simulink model "system_ID"  (R2023b)
settings: Solver=ode4  StartTime=0.0  StopTime=70  FixedStep=0.001  RelTol=1e-3
values from neighbouring files (symbols this model uses):
  Fc = 0.00040    (= 0.0004)    [MPC_casadi_block.m]    (also in continuous_cartpend.m; init_HAC_simulation.m; init_MPC.m; init_NMPC.m)
  g = [g; st_next - st_next_RK4]    [MPC_cartPend_casadi.m]    (also in MPC_cartPend_casadi_scaled.m; MPC_casadi_block.m; continuous_cartpend.m = 9.80665; init_HAC_simulation.m = 9.80665)
  I = 8.7395e-04    (= 0.00087395)    [MPC_casadi_block.m]    (also in continuous_cartpend.m = 0.0008739525; init_HAC_simulation.m = 0.0008739525; init_MPC.m = 0.0008739525; init_NMPC.m = 0.0008739525)
  init_angle = 180    [MPC_cartPend_casadi.m]    (also in init_HAC_simulation.m = deg2rad(initial_angle); init_MPC.m = -0.349065850399; init_NMPC.m = 3.14159265359; init_PID_cartpole.m = 0)
  kd = 0.000161    [MPC_casadi_block.m]    (also in continuous_cartpend.m; init_HAC_simulation.m; init_MPC.m; init_NMPC.m)
  kdr = 0.000001    (= 1e-06)    [MPC_casadi_block.m]    (also in continuous_cartpend.m; init_HAC_simulation.m; init_MPC.m; init_NMPC.m)
  kt = 150    [MPC_casadi_block.m]    (also in continuous_cartpend.m; init_HAC_simulation.m; init_MPC.m; init_NMPC.m)
  L = 0.1500    (= 0.15)    [MPC_casadi_block.m]    (also in continuous_cartpend.m; init_HAC_simulation.m; init_MPC.m; init_NMPC.m)
  m = 0.116527    [MPC_casadi_block.m]    (also in continuous_cartpend.m; init_HAC_simulation.m; init_MPC.m; init_NMPC.m)
libraries: simulink_extras x1
settings Model: Creator=doann  LastModifiedBy=doann
settings OptimizationCC: ReuseModelBlockBuffer=off

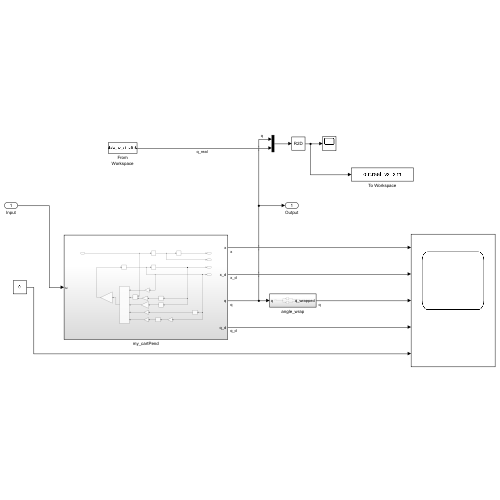
[thumbnail: Simulink's stored preview of the top-level diagram]
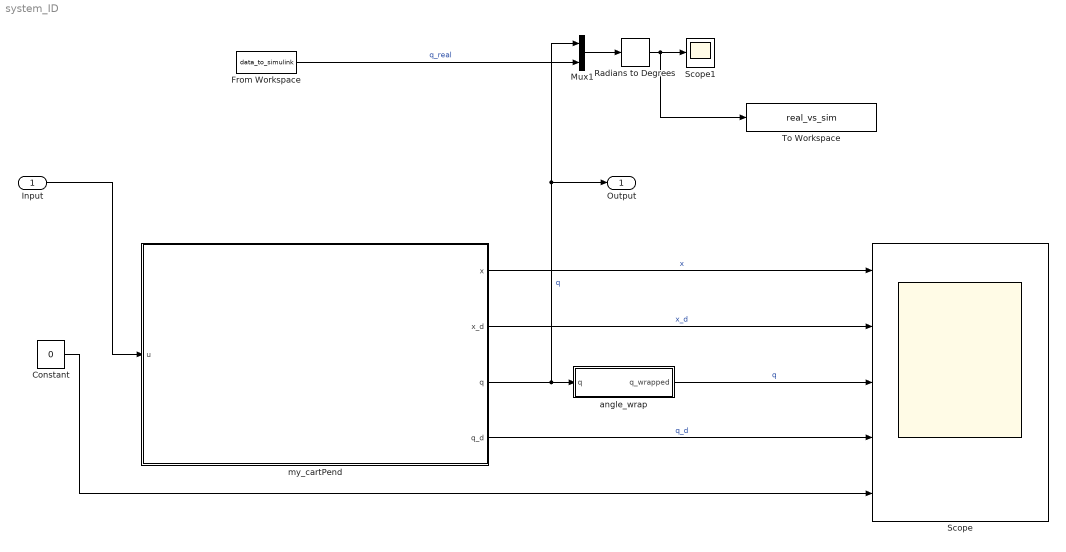
== system system_ID ==
  Input : Inport
  Constant : Constant  Value=0
  From Workspace : FromWorkspace  VariableName=data_to_simulink  OutputAfterFinalValue=Holding final value
  Mux1 : Mux  Inputs=2
  Radians to Degrees : simulink_extras/Transformations/Radians to Degrees
  Scope : Scope  NumInputPorts=5
  Scope1 : Scope
  To Workspace : ToWorkspace  VariableName=real_vs_sim  SaveFormat=Structure With Time  SampleTime=-1
  angle_wrap : Subsystem
  my_cartPend : Subsystem
  Output : Outport
  wires:
  Mux1/1 -> Radians to Degrees/1
  From Workspace/1 -> Mux1/2  "q_real"
  my_cartPend/3(q) -> Mux1/1, Output/1, angle_wrap/1(q)  "q"
  Constant/1 -> Scope/5
  angle_wrap/1(q_wrapped) -> Scope/3  "q"
  my_cartPend/1(x) -> Scope/1  "x"
  my_cartPend/2(x_d) -> Scope/2  "x_d"
  my_cartPend/4(q_d) -> Scope/4  "q_d"
  Input/1 -> my_cartPend/1(u)
  Radians to Degrees/1 -> To Workspace/1, Scope1/1

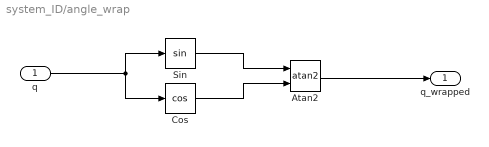
== system system_ID/angle_wrap ==
  q : Inport
  Atan2 : Trigonometry  Operator=atan2
  Cos : Trigonometry  Operator=cos
  Sin : Trigonometry
  q_wrapped : Outport
  wires:
  Cos/1 -> Atan2/2
  q/1 -> Sin/1, Cos/1
  Sin/1 -> Atan2/1
  Atan2/1 -> q_wrapped/1

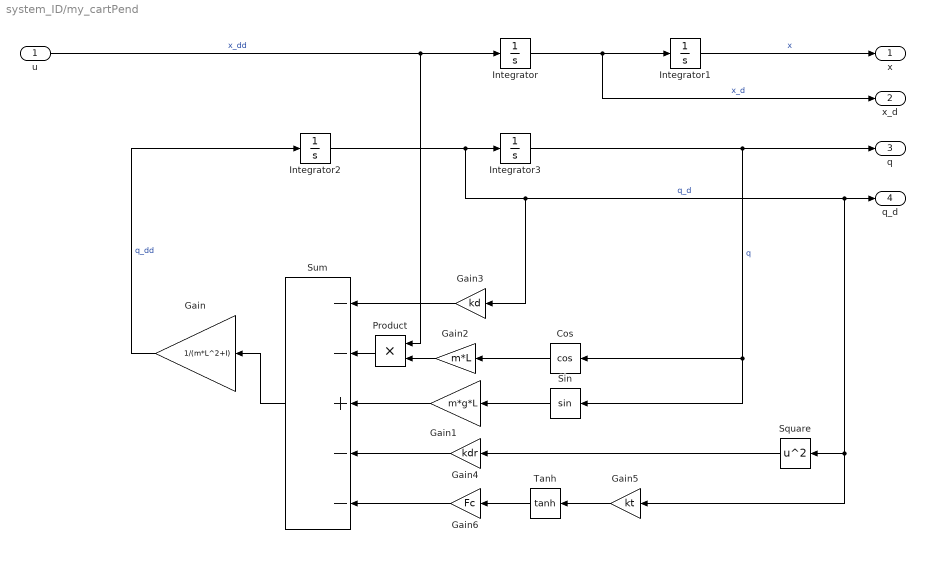
== system system_ID/my_cartPend ==
  u : Inport
  Cos : Trigonometry  Operator=cos
  Gain : Gain  Gain=1/(m*L^2+I)
  Gain1 : Gain  Gain=m*g*L
  Gain2 : Gain  Gain=m*L
  Gain3 : Gain  Gain=kd
  Gain4 : Gain  Gain=kdr
  Gain5 : Gain  Gain=kt
  Gain6 : Gain  Gain=Fc
  Integrator : Integrator
  Integrator1 : Integrator
  Integrator2 : Integrator
  Integrator3 : Integrator  InitialCondition=init_angle
  Product : Product
  Sin : Trigonometry
  Square : Math  Operator=square
  Sum : Sum  Inputs=--+--
  Tanh : Trigonometry  Operator=tanh
  x : Outport
  x_d : Outport  Port=2
  q : Outport  Port=3
  q_d : Outport  Port=4
  wires:
  u/1 -> Product/1, Integrator/1  "x_dd"
  Integrator/1 -> x_d/1, Integrator1/1  "x_d"
  Integrator1/1 -> x/1  "x"
  Integrator3/1 -> Sin/1, Cos/1, q/1  "q"
  Integrator2/1 -> Gain3/1, Gain5/1, Square/1, q_d/1, Integrator3/1  "q_d"
  Sin/1 -> Gain1/1
  Cos/1 -> Gain2/1
  Sum/1 -> Gain/1
  Gain/1 -> Integrator2/1  "q_dd"
  Gain1/1 -> Sum/3
  Gain3/1 -> Sum/1
  Gain2/1 -> Product/2
  Product/1 -> Sum/2
  Square/1 -> Gain4/1
  Tanh/1 -> Gain6/1
  Gain5/1 -> Tanh/1
  Gain4/1 -> Sum/4
  Gain6/1 -> Sum/5
